simulink model "Sirv2_0"  (R2023b)
settings: Solver=VariableStepAuto  StartTime=0.0  StopTime=10.0  RelTol=1e-3
values from neighbouring files (symbols this model uses):
  quadModel = block.DialogPrm(1).Data    [SirvDynamicsSFunction.m]    (also in Sirv_X.mat = ; Sirv_X_Backup.mat = )
undefined symbols (not defined in the file or in its folder): alpha, GOffset, Kdp, Kds, Kdt, Kdz, Kip, Kis, Kit, Kiz, Kpp, Kps, Kpt, Kpz, LSat, Ts, USat
libraries: simulink x4, bbblueActuatorLib x4, simulink_extras x2, bbblueSensorLib x1
settings Model: Creator=krali  LastModifiedBy=krali

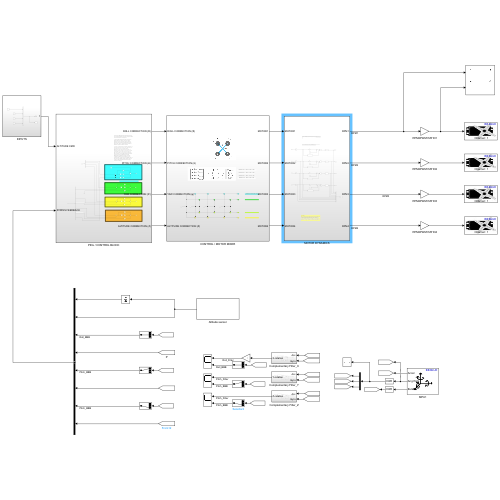
[thumbnail: Simulink's stored preview of the top-level diagram]
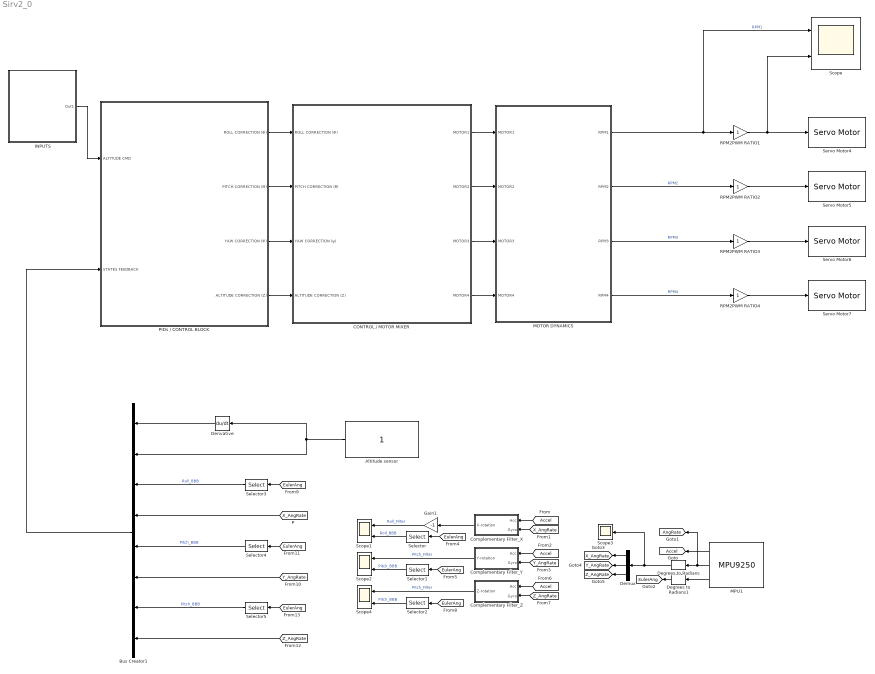
== system Sirv2_0 ==
  Altitude sensor : Constant
  Bus Creator1 : BusCreator  Inputs=8
  CONTROL / MOTOR MIXER : Subsystem
  Complementary Filter_X : Subsystem
  Complementary Filter_Y : Subsystem
  Complementary Filter_Z : Subsystem
  Degrees to Radians : simulink_extras/Transformations/Degrees to Radians
  Degrees to Radians1 : simulink_extras/Transformations/Degrees to Radians
  Demux : Demux  Outputs=3
  Derivative : Derivative
  Gain1 : Gain  Gain=-1
  INPUTS : Subsystem
  MOTOR DYNAMICS : Subsystem
  MPU1 : bbblueSensorLib/MPU9250  OperationMode=DMP  Accel=on  AngularRate=on  Ak8963Field=off  EulerAngles=on  Quat=off  AccelRange=2G  Acceldlpf=1  GyroRange=250 dps  Gyrodlpf=1  DmpOdr=200 Hz  SampleTime=0.003
  PIDs / CONTROL BLOCK : Subsystem
  RPM2PWM RATIO{1..4} (4 alike) : Gain
  Scope{,1..2,4} (4 alike) : Scope  NumInputPorts=2
  Scope3 : Scope
  Selector : Selector  InputPortWidth=3  IndexOptions=Index vector (dialog)  Indices=[2]  OutputSizes=1
  Selector1 : Selector  InputPortWidth=3  IndexOptions=Index vector (dialog)  Indices=[1]  OutputSizes=1
  Selector2 : Selector  InputPortWidth=3  IndexOptions=Index vector (dialog)  Indices=[3]  OutputSizes=1
  Selector3 : Selector  InputPortWidth=3  IndexOptions=Index vector (dialog)  Indices=[2]  OutputSizes=1
  Selector4 : Selector  InputPortWidth=3  IndexOptions=Index vector (dialog)  Indices=[1]  OutputSizes=1
  Selector5 : Selector  InputPortWidth=3  IndexOptions=Index vector (dialog)  Indices=[3]  OutputSizes=1
  Servo Motor{4..7} (4 alike) : bbblueActuatorLib/Servo Motor  channel=1  SimulateUsing=Code generation
  tag scope: Accel=global, AngRate=global, EulerAng=global, X_AngRate=global, Y_AngRate=global, Z_AngRate=global
  wires:
  PIDs / CONTROL BLOCK/1(ROLL CORRECTION (Φ)) -> CONTROL / MOTOR MIXER/1(ROLL CORRECTION (Φ))
  PIDs / CONTROL BLOCK/2(PITCH CORRECTION (Θ)) -> CONTROL / MOTOR MIXER/2(PITCH CORRECTION (θ))
  PIDs / CONTROL BLOCK/3(YAW CORRECTION (Ψ)) -> CONTROL / MOTOR MIXER/3(YAW CORRECTION (ψ))
  PIDs / CONTROL BLOCK/4(ALTITUDE CORRECTION (Ζ)) -> CONTROL / MOTOR MIXER/4(ALTITUDE CORRECTION (Z))
  CONTROL / MOTOR MIXER/1(MOTOR1) -> MOTOR DYNAMICS/1(MOTOR1)
  CONTROL / MOTOR MIXER/2(MOTOR2) -> MOTOR DYNAMICS/2(MOTOR2)
  CONTROL / MOTOR MIXER/3(MOTOR3) -> MOTOR DYNAMICS/3(MOTOR3)
  CONTROL / MOTOR MIXER/4(MOTOR4) -> MOTOR DYNAMICS/4(MOTOR4)
  INPUTS/1(Out1) -> PIDs / CONTROL BLOCK/1(ALTITUDE CMD)
  MOTOR DYNAMICS/1(RPM1) -> Scope/1, RPM2PWM RATIO1/1  "RPM1"
  MOTOR DYNAMICS/2(RPM2) -> RPM2PWM RATIO2/1  "RPM2"
  MOTOR DYNAMICS/3(RPM3) -> RPM2PWM RATIO3/1  "RPM3"
  MOTOR DYNAMICS/4(RPM4) -> RPM2PWM RATIO4/1  "RPM4"
  RPM2PWM RATIO1/1 -> Servo Motor4/1, Scope/2
  RPM2PWM RATIO2/1 -> Servo Motor5/1
  RPM2PWM RATIO3/1 -> Servo Motor6/1
  RPM2PWM RATIO4/1 -> Servo Motor7/1
  Bus Creator1/1 -> PIDs / CONTROL BLOCK/2(STATES FEEDBACK)
  Altitude sensor/1 -> Bus Creator1/2, Derivative/1
  Derivative/1 -> Bus Creator1/1
  MPU1/3 -> Degrees to Radians1/1
  Degrees to Radians1/1 -> [EulerAng]
  Demux/2 -> [Y_AngRate]
  Degrees to Radians/1 -> Demux/1, Scope3/1
  Demux/3 -> [Z_AngRate]
  MPU1/2 -> [AngRate], Degrees to Radians/1
  Demux/1 -> [X_AngRate]
  MPU1/1 -> [Accel]
  Complementary Filter_X/1(X-rotation) -> Gain1/1
  Gain1/1 -> Scope1/1  "Roll_Filter"
  [Accel] -> Complementary Filter_Y/1(Acc)
  [EulerAng] -> Selector/1
  [EulerAng] -> Selector1/1
  Selector/1 -> Scope1/2  "Roll_BBB"
  [Accel] -> Complementary Filter_X/1(Acc)
  [Y_AngRate] -> Complementary Filter_Y/2(Gyro)
  [X_AngRate] -> Complementary Filter_X/2(Gyro)
  Complementary Filter_Y/1(Y-rotation) -> Scope2/1  "Pitch_Filter"
  Selector1/1 -> Scope2/2  "Pitch_BBB"
  [EulerAng] -> Selector2/1
  [Z_AngRate] -> Complementary Filter_Z/2(Gyro)
  Selector2/1 -> Scope4/2  "Pitch_BBB"
  [Accel] -> Complementary Filter_Z/1(Acc)
  Complementary Filter_Z/1(Z-rotation) -> Scope4/1  "Pitch_Filter"
  Selector3/1 -> Bus Creator1/3  "Roll_BBB"
  [EulerAng] -> Selector3/1
  [X_AngRate] -> Bus Creator1/4
  [Y_AngRate] -> Bus Creator1/6
  Selector4/1 -> Bus Creator1/5  "Pitch_BBB"
  [EulerAng] -> Selector4/1
  Selector5/1 -> Bus Creator1/7  "Pitch_BBB"
  [EulerAng] -> Selector5/1
  [Z_AngRate] -> Bus Creator1/8

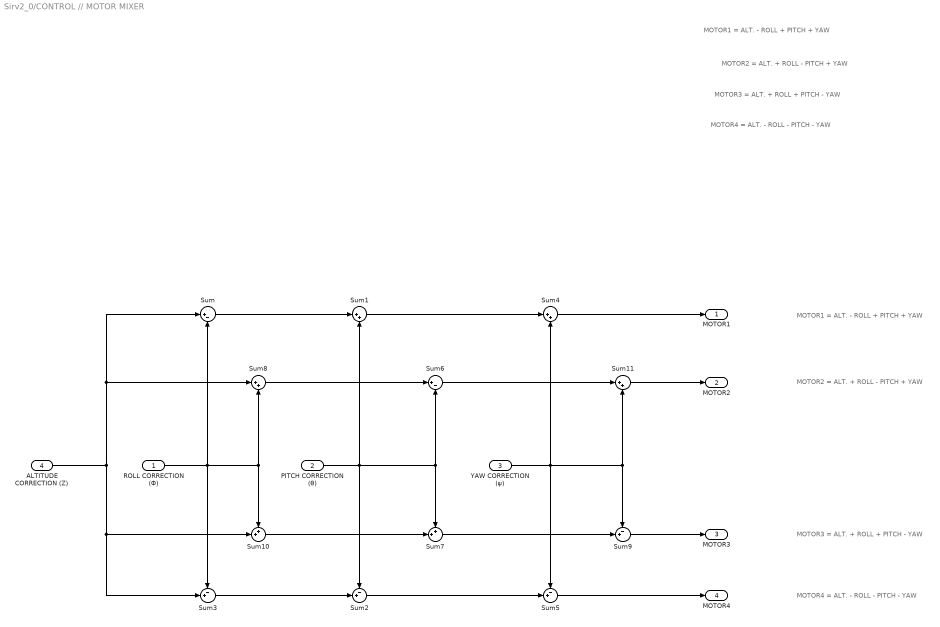
== system Sirv2_0/CONTROL // MOTOR MIXER ==
  note: MOTOR1 = ALT. - ROLL + PITCH + YAW
  note: MOTOR2 = ALT. + ROLL - PITCH + YAW
  note: MOTOR3 = ALT. + ROLL + PITCH - YAW
  note: MOTOR4 = ALT. - ROLL - PITCH - YAW
  note: MOTOR1 = ALT. - ROLL + PITCH + YAW
  note: MOTOR2 = ALT. + ROLL - PITCH + YAW
  note: MOTOR3 = ALT. + ROLL + PITCH - YAW
  note: MOTOR4 = ALT. - ROLL - PITCH - YAW
  ROLL CORRECTION (Φ) : Inport
  PITCH CORRECTION (θ) : Inport  Port=2
  YAW CORRECTION (ψ) : Inport  Port=3
  ALTITUDE CORRECTION (Z) : Inport  Port=4
  Sum : Sum  Inputs=|+-
  Sum{1,4,8,11} (4 alike) : Sum  Inputs=|++
  Sum10 : Sum  Inputs=++|
  Sum{2..3,5,9} (4 alike) : Sum  Inputs=-+|
  Sum6 : Sum  Inputs=|+-
  Sum7 : Sum  Inputs=++|
  MOTOR1 : Outport
  MOTOR2 : Outport  Port=2
  MOTOR3 : Outport  Port=3
  MOTOR4 : Outport  Port=4
  wires:
  PITCH CORRECTION (θ)/1 -> Sum6/2, Sum7/1, Sum2/1, Sum1/2
  ROLL CORRECTION (Φ)/1 -> Sum8/2, Sum10/1, Sum3/1, Sum/2
  ALTITUDE CORRECTION (Z)/1 -> Sum8/1, Sum/1, Sum10/2, Sum3/2
  Sum/1 -> Sum1/1
  Sum1/1 -> Sum4/1
  Sum3/1 -> Sum2/2
  Sum2/1 -> Sum5/2
  Sum4/1 -> MOTOR1/1
  Sum5/1 -> MOTOR4/1
  Sum10/1 -> Sum7/2
  Sum7/1 -> Sum9/2
  Sum9/1 -> MOTOR3/1
  Sum8/1 -> Sum6/1
  Sum11/1 -> MOTOR2/1
  Sum6/1 -> Sum11/1
  YAW CORRECTION (ψ)/1 -> Sum5/1, Sum9/1, Sum11/2, Sum4/2

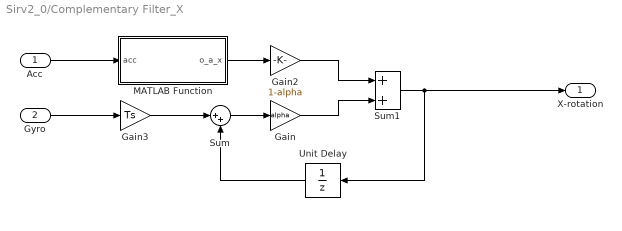
== system Sirv2_0/Complementary Filter_X ==
  Acc : Inport
  Gyro : Inport  Port=2
  Gain : Gain  Gain=alpha
  Gain2 : Gain  Gain=1-alpha
  Gain3 : Gain  Gain=Ts
  MATLAB Function : MATLAB Function  TreatAsAtomicUnit=on
  Sum : Sum  Inputs=|++
  Sum1 : Sum
  Unit Delay : UnitDelay  SampleTime=-1  HasFrameUpgradeWarning=on
  X-rotation : Outport
  wires:
  MATLAB Function/1(o_a_x) -> Gain2/1
  Gain/1 -> Sum1/2
  Sum/1 -> Gain/1
  Acc/1 -> MATLAB Function/1(acc)
  Gain2/1 -> Sum1/1
  Unit Delay/1 -> Sum/2
  Gain3/1 -> Sum/1
  Gyro/1 -> Gain3/1
  Sum1/1 -> X-rotation/1, Unit Delay/1

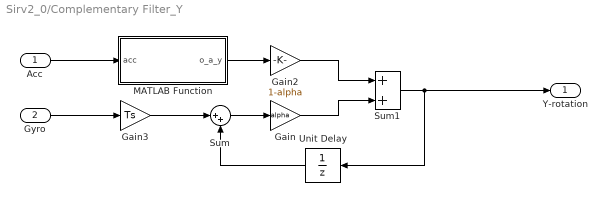
== system Sirv2_0/Complementary Filter_Y ==
  Acc : Inport
  Gyro : Inport  Port=2
  Gain : Gain  Gain=alpha
  Gain2 : Gain  Gain=1-alpha
  Gain3 : Gain  Gain=Ts
  MATLAB Function : MATLAB Function  TreatAsAtomicUnit=on
  Sum : Sum  Inputs=|++
  Sum1 : Sum
  Unit Delay : UnitDelay  SampleTime=-1  HasFrameUpgradeWarning=on
  Y-rotation : Outport
  wires:
  MATLAB Function/1(o_a_y) -> Gain2/1
  Gain/1 -> Sum1/2
  Sum/1 -> Gain/1
  Acc/1 -> MATLAB Function/1(acc)
  Gain2/1 -> Sum1/1
  Unit Delay/1 -> Sum/2
  Gain3/1 -> Sum/1
  Gyro/1 -> Gain3/1
  Sum1/1 -> Y-rotation/1, Unit Delay/1

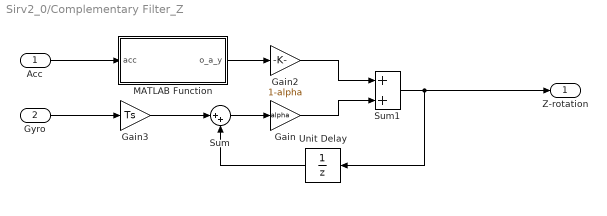
== system Sirv2_0/Complementary Filter_Z ==
  Acc : Inport
  Gyro : Inport  Port=2
  Gain : Gain  Gain=alpha
  Gain2 : Gain  Gain=1-alpha
  Gain3 : Gain  Gain=Ts
  MATLAB Function : MATLAB Function  TreatAsAtomicUnit=on
  Sum : Sum  Inputs=|++
  Sum1 : Sum
  Unit Delay : UnitDelay  SampleTime=-1  HasFrameUpgradeWarning=on
  Z-rotation : Outport
  wires:
  MATLAB Function/1(o_a_y) -> Gain2/1
  Gain/1 -> Sum1/2
  Sum/1 -> Gain/1
  Acc/1 -> MATLAB Function/1(acc)
  Gain2/1 -> Sum1/1
  Unit Delay/1 -> Sum/2
  Gain3/1 -> Sum/1
  Gyro/1 -> Gain3/1
  Sum1/1 -> Z-rotation/1, Unit Delay/1

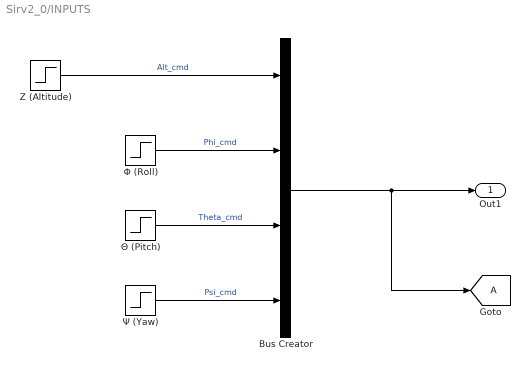
== system Sirv2_0/INPUTS ==
  Bus Creator : BusCreator  Inputs=4
  Goto : Goto  TagVisibility=global
  Z (Altitude) : Step  SampleTime=0
  Θ (Pitch) : Step  SampleTime=0
  Φ (Roll) : Step  SampleTime=0
  Ψ (Yaw) : Step  SampleTime=0
  Out1 : Outport
  wires:
  Z (Altitude)/1 -> Bus Creator/1  "Alt_cmd"
  Ψ (Yaw)/1 -> Bus Creator/4  "Psi_cmd"
  Φ (Roll)/1 -> Bus Creator/2  "Phi_cmd"
  Bus Creator/1 -> Goto/1, Out1/1
  Θ (Pitch)/1 -> Bus Creator/3  "Theta_cmd"

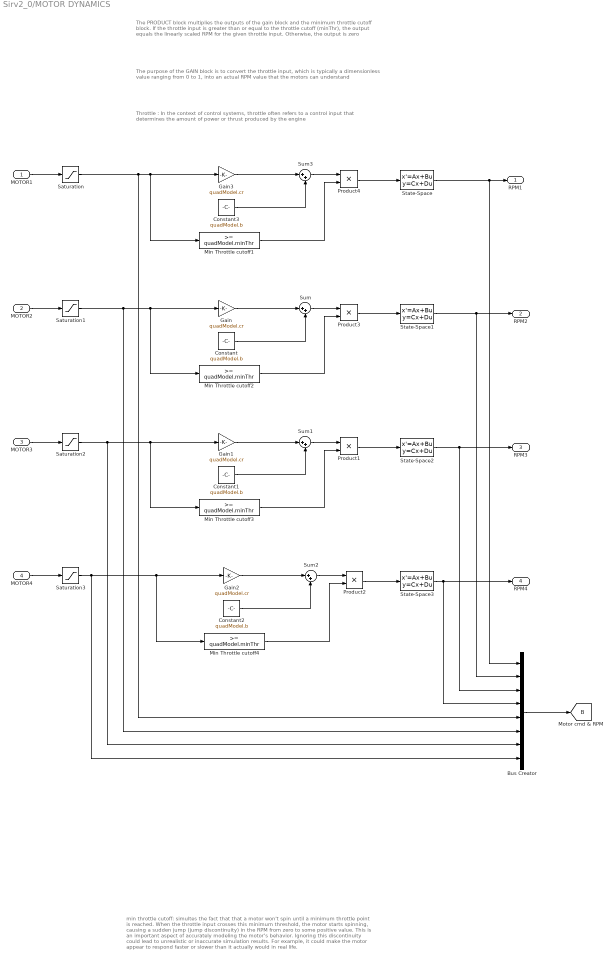
== system Sirv2_0/MOTOR DYNAMICS ==
  note: Throttle : In the context of control systems, throttle often refers to a control input that determines the amount of power or thrust produced by the engine
  note: The PRODUCT block multiplies the outputs of the gain block and the minimum throttle cutoff block. If the throttle input is greater than or equal to the throttle cutoff (minThr), the output equals the linearly scaled RPM for the given throttle input. Otherwise, the output is zero
  note: The purpose of the GAIN block is to convert the throttle input, which is typically a dimensionless value ranging from 0 to 1, into an actual RPM value that the motors can understand
  note: min throttle cutoff: simultes the fact that that a motor won't spin until a minimum throttle point is reached.
      |
      | When the throttle input crosses this minimum threshold, the motor starts spinning, causing a sudden jump (jump discontinuity) in the RPM from zero to some positive value. This is an important aspect of accurately modeling the motor’s behavior. Ignoring this discontinuity could lead to unrealistic or inaccurate simulation results. For example, it could make the motor appear to respond faster or slower than it actually would in real life.
  MOTOR1 : Inport
  MOTOR2 : Inport  Port=2
  MOTOR3 : Inport  Port=3
  MOTOR4 : Inport  Port=4
  Bus Creator : BusCreator  Inputs=8
  Constant{,1..3} (4 alike) : Constant  Value=quadModel.b
  Gain{,1..3} (4 alike) : Gain  Gain=quadModel.cr
  Min Throttle cutoff{1..4} (4 alike) : simulink/Logic and Bit Operations/Compare To Constant  relop=>=  const=quadModel.minThr  OutDataTypeStr=boolean
  Product{1..4} (4 alike) : Product
  Saturation{,1..3} (4 alike) : Saturate
  State-Space{,1..3} (4 alike) : StateSpace  InitialCondition=0
  Sum{,1..3} (4 alike) : Sum  Inputs=|++
  RPM1 : Outport
  RPM2 : Outport  Port=2
  RPM3 : Outport  Port=3
  RPM4 : Outport  Port=4
  tag scope: B=global
  wires:
  Product1/1 -> State-Space2/1
  MOTOR4/1 -> Saturation3/1
  State-Space3/1 -> Bus Creator/4, RPM4/1
  State-Space2/1 -> Bus Creator/3, RPM3/1
  MOTOR2/1 -> Saturation1/1
  State-Space/1 -> Bus Creator/1, RPM1/1
  MOTOR3/1 -> Saturation2/1
  State-Space1/1 -> Bus Creator/2, RPM2/1
  MOTOR1/1 -> Saturation/1
  Product4/1 -> State-Space/1
  Min Throttle cutoff2/1 -> Product3/2
  Saturation1/1 -> Bus Creator/6, Gain/1, Min Throttle cutoff2/1
  Sum/1 -> Product3/1
  Gain/1 -> Sum/1
  Product3/1 -> State-Space1/1
  Constant/1 -> Sum/2
  Constant1/1 -> Sum1/2
  Gain1/1 -> Sum1/1
  Sum1/1 -> Product1/1
  Saturation2/1 -> Bus Creator/7, Gain1/1, Min Throttle cutoff3/1
  Min Throttle cutoff3/1 -> Product1/2
  Constant2/1 -> Sum2/2
  Gain2/1 -> Sum2/1
  Sum2/1 -> Product2/1
  Saturation3/1 -> Bus Creator/8, Gain2/1, Min Throttle cutoff4/1
  Min Throttle cutoff4/1 -> Product2/2
  Product2/1 -> State-Space3/1
  Constant3/1 -> Sum3/2
  Gain3/1 -> Sum3/1
  Sum3/1 -> Product4/1
  Saturation/1 -> Bus Creator/5, Gain3/1, Min Throttle cutoff1/1
  Min Throttle cutoff1/1 -> Product4/2
  Bus Creator/1 -> [B]

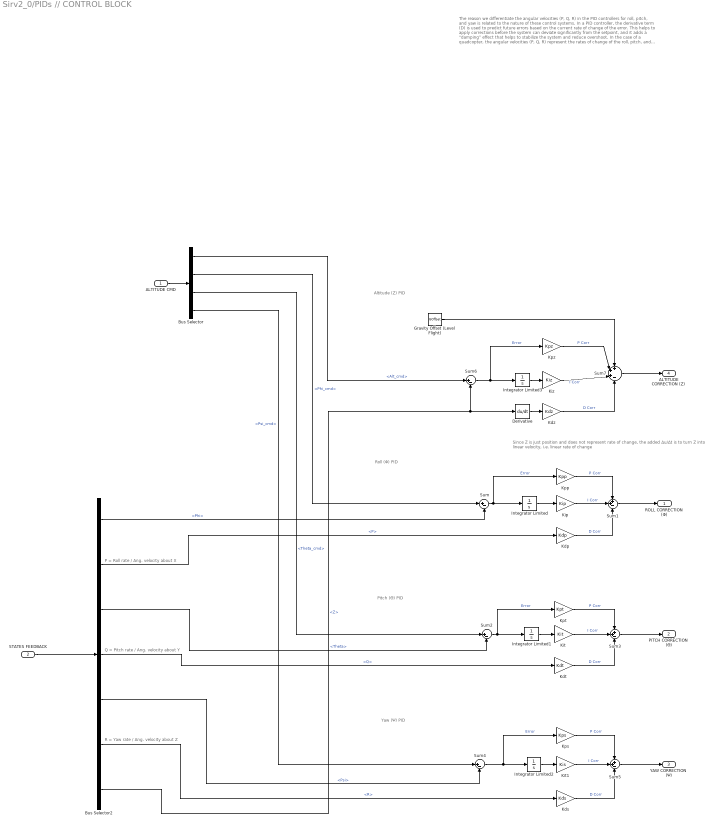
== system Sirv2_0/PIDs // CONTROL BLOCK ==
  note: Since Z is just position and does not represent rate of change, the added Δu/Δt is to turn Z into linear velocity, i.e. linear rate of change
  note: The reason we differentiate the angular velocities (P, Q, R) in the PID controllers for roll, pitch, and yaw is related to the nature of these control systems.
      | In a PID controller, the derivative term (D) is used to predict future errors based on the current rate of change of the error. This helps to apply corrections before the system can deviate significantly from the setpoint, and it adds a “damping” effect that helps to stabilize the system and reduce overshoot.
      | In the case of a quadcopter, the angular velocities (P, Q, R) represent the rates of change of the roll, pitch, and yaw angles (Phi, Theta, Psi), respectively. By differentiating these values, the PID controller can effectively “predict” changes in the roll, pitch, and yaw angles based on their current rates of change. This allows the controller to apply corrections proactively, which can result in more stable and responsive control.
      | On the other hand, the altitude PID controller differentiates the altitude (Z) because it’s directly controlling the altitude of the quadcopter, not an angular quantity. The derivative of the altitude gives the rate of change of altitude (vertical velocity), which can be used to predict future altitude errors and apply corrections accordingly.
  note: R = Yaw rate / Ang. velocity about Z
  note: Yaw (Ψ) PID
  note: Pitch (Θ) PID
  note: Roll (Φ) PID
  note: Altitude (Z) PID
  note: Q = Pitch rate / Ang. velocity about Y
  note: P = Roll rate / Ang. velocity about X
  ALTITUDE CMD : Inport
  STATES FEEDBACK : Inport  Port=2
  Bus Selector : BusSelector  OutputSignals=Alt_cmd,Phi_cmd,Theta_cmd,Psi_cmd
  Bus Selector2 : BusSelector  OutputSignals=Phi,P,Theta,Q,Psi,R,Z
  Derivative : Derivative
  Gravity Offset (Level Flight) : Constant  Value=GOffset
  Integrator Limited{,1..3} (4 alike) : Integrator  LimitOutput=on  UpperSaturationLimit=USat  LowerSaturationLimit=LSat
  Kdp : Gain  Gain=Kdp
  Kds : Gain  Gain=Kds
  Kdt : Gain  Gain=Kdt
  Kdz : Gain  Gain=Kdz
  Kip : Gain  Gain=Kip
  Kit : Gain  Gain=Kit
  Kit1 : Gain  Gain=Kis
  Kiz : Gain  Gain=Kiz
  Kpp : Gain  Gain=Kpp
  Kps : Gain  Gain=Kps
  Kpt : Gain  Gain=Kpt
  Kpz : Gain  Gain=Kpz
  Sum{,2,4,6} (4 alike) : Sum  Inputs=|+-
  Sum1 : Sum  Inputs=++-
  Sum3 : Sum  Inputs=++-
  Sum5 : Sum  Inputs=++-
  Sum7 : Sum  Inputs=+++-
  ROLL CORRECTION (Φ) : Outport
  PITCH CORRECTION (Θ) : Outport  Port=2
  YAW CORRECTION (Ψ) : Outport  Port=3
  ALTITUDE CORRECTION (Ζ) : Outport  Port=4
  wires:
  ALTITUDE CMD/1 -> Bus Selector/1
  Sum/1 -> Kpp/1, Integrator Limited/1  "Error"
  Sum1/1 -> ROLL CORRECTION (Φ)/1
  Kip/1 -> Sum1/2  "I Corr"
  Kdp/1 -> Sum1/3  "D Corr"
  Integrator Limited/1 -> Kip/1
  Kpp/1 -> Sum1/1  "P Corr"
  STATES FEEDBACK/1 -> Bus Selector2/1
  Sum2/1 -> Integrator Limited1/1, Kpt/1  "Error"
  Sum3/1 -> PITCH CORRECTION (Θ)/1
  Kpt/1 -> Sum3/1  "P Corr"
  Integrator Limited1/1 -> Kit/1
  Kdt/1 -> Sum3/3  "D Corr"
  Kit/1 -> Sum3/2  "I Corr"
  Bus Selector/3 -> Sum2/1  "<Theta_cmd>"
  Bus Selector/2 -> Sum/1  "<Phi_cmd>"
  Sum5/1 -> YAW CORRECTION (Ψ)/1
  Bus Selector/4 -> Sum4/1  "<Psi_cmd>"
  Integrator Limited2/1 -> Kit1/1
  Kds/1 -> Sum5/3  "D Corr"
  Kps/1 -> Sum5/1  "P Corr"
  Kit1/1 -> Sum5/2  "I Corr"
  Sum4/1 -> Kps/1, Integrator Limited2/1  "Error"
  Bus Selector/1 -> Sum6/1  "<Alt_cmd>"
  Kpz/1 -> Sum7/2  "P Corr"
  Sum6/1 -> Kpz/1, Integrator Limited3/1  "Error"
  Sum7/1 -> ALTITUDE CORRECTION (Ζ)/1
  Gravity Offset (Level Flight)/1 -> Sum7/1
  Kiz/1 -> Sum7/3  "I Corr"
  Kdz/1 -> Sum7/4  "D Corr"
  Derivative/1 -> Kdz/1
  Integrator Limited3/1 -> Kiz/1
  Bus Selector2/1 -> Sum/2  "<Phi>"
  Bus Selector2/2 -> Kdp/1  "<P>"
  Bus Selector2/3 -> Sum2/2  "<Theta>"
  Bus Selector2/4 -> Kdt/1  "<Q>"
  Bus Selector2/5 -> Sum4/2  "<Psi>"
  Bus Selector2/6 -> Kds/1  "<R>"
  Bus Selector2/7 -> Sum6/2, Derivative/1  "<Z>"

== matlab function Sirv2_0/Complementary Filter_Z/MATLAB Function ==
  data: acc input; o_a_y output
function o_a_y = fcn(acc)

acc_y = acc(2);
acc_z = acc(3);

o_a_y = atan(acc_y/acc_z);

end

== matlab function Sirv2_0/Complementary Filter_X/MATLAB Function ==
  data: acc input; o_a_x output
function o_a_x = fcn(acc)

acc_x = acc(1);
acc_z = acc(3);

o_a_x = atan(acc_x/acc_z);

end

== matlab function Sirv2_0/Complementary Filter_Y/MATLAB Function ==
  data: acc input; o_a_y output
function o_a_y = fcn(acc)

acc_y = acc(2);
acc_z = acc(3);

o_a_y = atan(acc_y/acc_z);

end
